simulink model "XZSim"  (R2023b)
settings: Solver=VariableStepAuto  StartTime=0.0  StopTime=60  RelTol=1e-8
undefined symbols (not defined in the file): K, theta_dot_ref, theta_ref, x_dot_ref, x_ref
libraries: simulink_extras x2
settings Model: Creator=leand  LastModifiedBy=leand

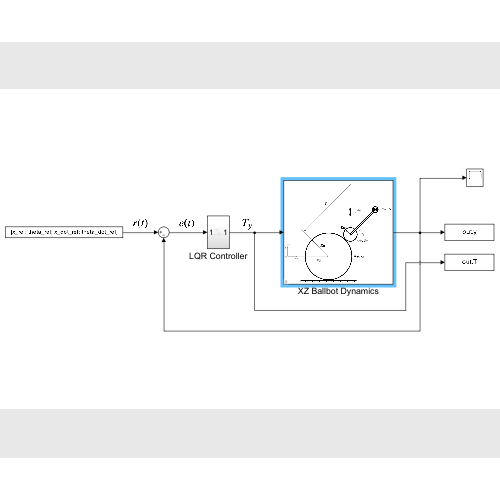
[thumbnail: Simulink's stored preview of the top-level diagram]
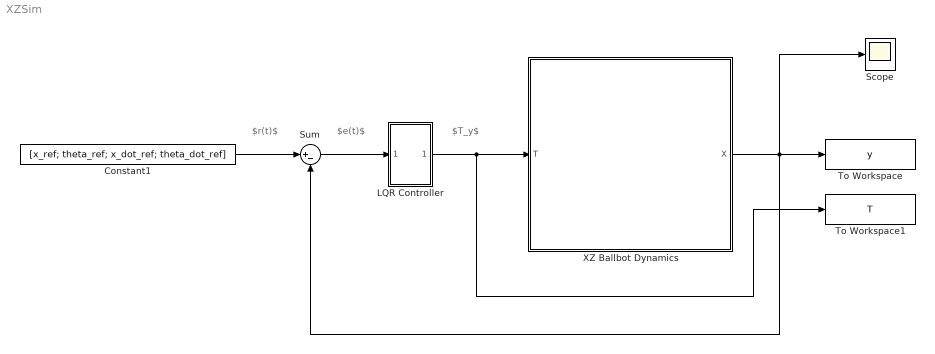
== system XZSim ==
  note: $T_y$
  note: $e(t)$
  note: $r(t)$
  Constant1 : Constant  Value=[x_ref; theta_ref; x_dot_ref; theta_dot_ref]
  LQR Controller : Subsystem
  Scope : Scope
  Sum : Sum  Inputs=|+-
  To Workspace : ToWorkspace  VariableName=y  SaveFormat=Timeseries  SampleTime=-1
  To Workspace1 : ToWorkspace  VariableName=T  SaveFormat=Timeseries  SampleTime=-1
  XZ Ballbot Dynamics : Subsystem  mask{x_0=-1, x_dot_0=0, theta_0=0, theta_dot_0=0}
      mask prompts: x_0 "Insert Ball initial position (m)"; x_dot_0 "Insert Ball initial velocity (m/s)"; theta_0 "Insert Robot initial Pitch Angle (°)"; theta_dot_0 "Insert Robot initial Pitch Angle Rate (º/s)"
      mask Display: image('XZ_a.png');
  wires:
  XZ Ballbot Dynamics/1(X) -> Scope/1, Sum/2, To Workspace/1
  Constant1/1 -> Sum/1
  LQR Controller/1(Out1) -> XZ Ballbot Dynamics/1(T), To Workspace1/1
  Sum/1 -> LQR Controller/1(In1)

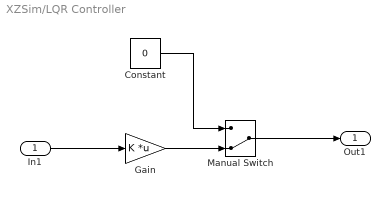
== system XZSim/LQR Controller ==
  In1 : Inport
  Constant : Constant  Value=0
  Gain : Gain  Gain=K  Multiplication=Matrix(K*u)
  Manual Switch : ManualSwitch  CurrentSetting=0
  Out1 : Outport
  wires:
  Gain/1 -> Manual Switch/2
  Constant/1 -> Manual Switch/1
  Manual Switch/1 -> Out1/1
  In1/1 -> Gain/1

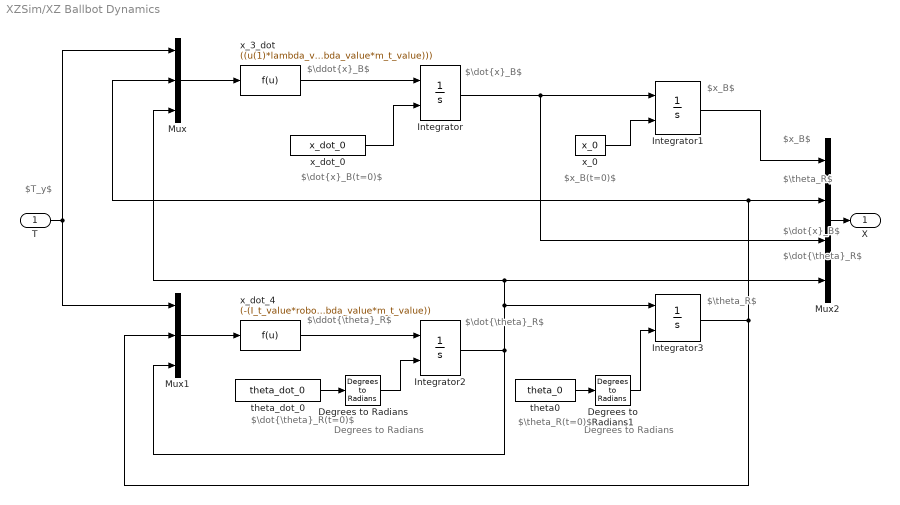
== system XZSim/XZ Ballbot Dynamics ==
  note: $x_B(t=0)$
  note: $\dot{\theta}_R(t=0)$
  note: Degrees to
      | Radians
  note: $T_y$
  note: $\ddot{\theta}_R$
  note: $\ddot{x}_B$
  note: $\dot{x}_B$
  note: $x_B$
  note: $\dot{\theta}_R$
  note: $\theta_R$
  note: $x_B$
  note: $\dot{x}_B$
  note: $\theta_R$
  note: $\dot{\theta}_R$
  note: Degrees to
      | Radians
  note: $\theta_R(t=0)$
  note: $\dot{x}_B(t=0)$
  T : Inport
  Degrees to Radians : simulink_extras/Transformations/Degrees to Radians
  Degrees to Radians1 : simulink_extras/Transformations/Degrees to Radians
  Integrator{,1..3} (4 alike) : Integrator  InitialConditionSource=external
  Mux : Mux  Inputs=3
  Mux1 : Mux  Inputs=3
  Mux2 : Mux
  theta0 : Constant  Value=theta_0
  theta_dot_0 : Constant  Value=theta_dot_0
  x_0 : Constant  Value=x_0
  x_3_dot : Fcn  Expr=((u(1)*lambda_value)+(robot.R_b*u(1)*gamma_value*cos(u(2)))-(robot.I_w*robot.R_b*u(1)*eta_value)+(robot.R_w*gamma_value*lambda_value*u(3)^2*sin(u(2)))-(robot.R_w*g_value*gamma_value^2*cos(u(2))*sin(u(2)))+(robot.I_w*robot.R_w*eta_value*g_value*gamma_value*sin(u(2))))/(robot.R_w*((-robot.I_w^2*eta_value^2)+(2*robot.I_w*eta_value*gamma_value*cos(u(2)))-(gamma_value^2*cos(u(2))^2)+(I_t_value*lambda_value)+(lambda_value*m_t_value)))
  x_dot_0 : Constant  Value=x_dot_0
  x_dot_4 : Fcn  Expr=(-(I_t_value*robot.R_b*u(1))+(robot.I_w*u(1)*eta_value)-(robot.R_b*u(1)*m_t_value)-(u(1)*gamma_value*cos(u(2)))-(robot.R_w*gamma_value^2*u(3)^2*cos(u(2))*sin(u(2)))+(I_t_value*robot.R_w*g_value*gamma_value*sin(u(2)))+(robot.R_w*g_value*gamma_value*m_t_value*sin(u(2)))+(robot.I_w*robot.R_w*eta_value*gamma_value*u(3)^2*sin(u(2))))/(robot.R_w*((-robot.I_w^2*eta_value^2)+(2*robot.I_w*eta_value*gamma_value*cos(u(2)))-(gamma_value^2*cos(u(2))^2)+(I_t_value*lambda_value)+lambda_value*m_t_value))
  X : Outport
  wires:
  x_3_dot/1 -> Integrator/1
  Integrator/1 -> Mux2/3, Integrator1/1
  Integrator2/1 -> Mux2/4, Mux/3, Integrator3/1, Mux1/3
  Integrator1/1 -> Mux2/1
  x_dot_4/1 -> Integrator2/1
  Mux/1 -> x_3_dot/1
  Mux1/1 -> x_dot_4/1
  Integrator3/1 -> Mux2/2, Mux/2, Mux1/2
  T/1 -> Mux/1, Mux1/1
  x_0/1 -> Integrator1/2
  x_dot_0/1 -> Integrator/2
  Degrees to Radians/1 -> Integrator2/2
  theta_dot_0/1 -> Degrees to Radians/1
  Degrees to Radians1/1 -> Integrator3/2
  theta0/1 -> Degrees to Radians1/1
  Mux2/1 -> X/1
